simulink model "test_seven_level_flying_cap_leg"  (R2017b)
settings: Solver=ode4  StartTime=0.0  StopTime=0.04  FixedStep=1e-6  MaxStep=1e-4  RelTol=1e-3
libraries: powerlib x10, typhoonHILlib x1
settings Model: Creator=Marcos  LastModifiedBy=Marcos

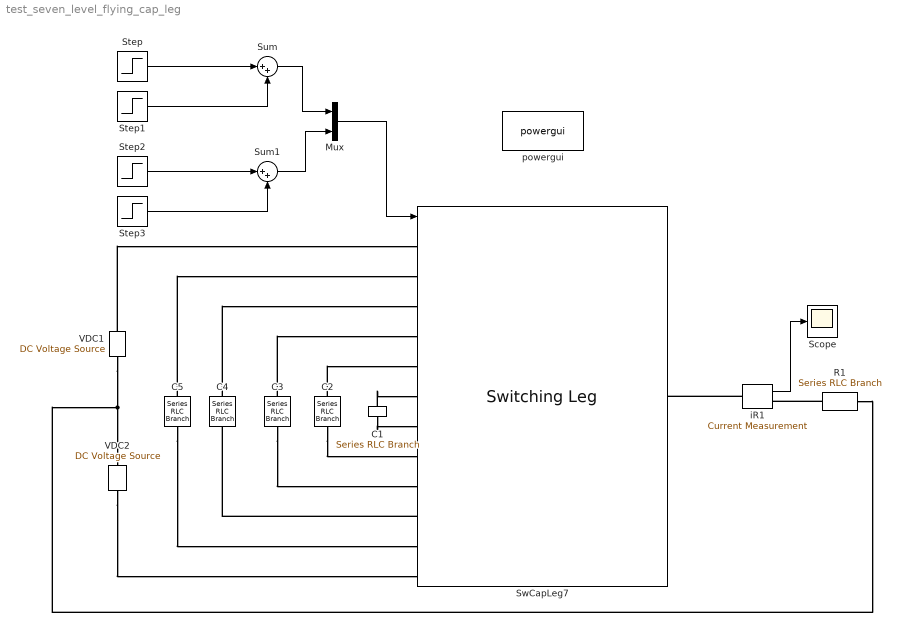
== system test_seven_level_flying_cap_leg ==
  C1 : powerlib/Elements/Series RLC Branch  LConnTagsString=__new0  RConnTagsString=__new0  BranchType=C  Resistance=1  Inductance=1e-3  SetiL0=off  InitialCurrent=0  Capacitance=3e-3  Setx0=on  InitialVoltage=0  Measurements=None
  C{2..5} (4 alike) : powerlib/Elements/Series RLC Branch  LConnTagsString=__new0  RConnTagsString=__new0  BranchType=C  Resistance=1  Inductance=1e-3  SetiL0=off  InitialCurrent=0  Capacitance=1e-3  Setx0=on  InitialVoltage=0  Measurements=None
  Mux : Mux  Inputs=2
  R1 : powerlib/Elements/Series RLC Branch  LConnTagsString=__new0  RConnTagsString=__new0  BranchType=R  Resistance=10  Inductance=1e-3  SetiL0=off  InitialCurrent=0  Capacitance=1e-6  Setx0=off  InitialVoltage=0  Measurements=None
  Scope : Scope
  Step : Step  Time=0  Before=[0 0 0 0 0 0]  After=[0 0 0 0 0 1]  SampleTime=0
  Step1 : Step  Time=0.02  Before=[0 0 0 0 0 0]  After=[1 1 1 1 1 0]  SampleTime=0
  Step2 : Step  Time=0  Before=[0 0 0 0 0 0]  After=[0 1 1 1 1 1]  SampleTime=0
  Step3 : Step  Time=0.02  Before=[0 0 0 0 0 0]  After=[0 -1 -1 -1 -1 -1]  SampleTime=0
  Sum : Sum  Inputs=|++
  Sum1 : Sum  Inputs=|++
  SwCapLeg7 : typhoonHILlib/Switching Leg  LegType=Flying Capacitor  Ttype=on  FCLevels=Seven-level  s1_logic=Active-high  s2_logic=Active-high  s3_logic=Active-high  s4_logic=Active-high  s5_logic=Active-high  s6_logic=Active-high  s7_logic=Active-high  s8_logic=Active-high  s9_logic=Active-high  s10_logic=Active-high  s11_logic=Active-high  s12_logic=Active-high  s13_logic=Active-high  s14_logic=Active-high  s15_logic=Active-high  s16_logic=Active-high  di_s1=1  di_s2=2  di_s3=3  di_s4=4  di_s5=5  di_s6=6  di_s7=7  di_s8=8  di_s9=9  di_s10=10  di_s11=11  di_s12=12  di_s13=13  di_s14=14  di_s15=15  di_s16=16  v_s1=off  v_s2=off  v_s3=off  v_s4=off  v_s5=off  v_s6=off  v_s7=off  v_s8=off  v_s9=off  v_s10=off  v_s11=off  v_s12=off  v_s13=off  v_s14=off  v_s15=off  v_s16=off  i_s1=off  i_s2=off  i_s3=off  i_s4=off  i_s5=off  i_s6=off  i_s7=off  i_s8=off  i_s9=off  i_s10=off  i_s11=off  i_s12=off  i_s13=off  i_s14=off  i_s15=off  i_s16=off  r_on=0.001  v_f=0  r_s=1e4  c_s=inf  toggle_init=on  toggle_draw=on  model_loaded=off  old_pat=typhoonPatterns/FC Leg (7-level)  old_size=250,380
      settings: SourceProductName=Typhoon HIL
  VDC1 : powerlib/Electrical Sources/DC Voltage Source  Amplitude=100  Measurements=None
  VDC2 : powerlib/Electrical Sources/DC Voltage Source  Amplitude=100  Measurements=None
  iR1 : powerlib/Measurements/Current Measurement  PhasorSimulation=off  OutputType=Complex  PSBequivalent=0
  powergui : powerlib/powergui  Priority=1  SimulationMode=Continuous  SampleTime=10e-6  frequency=60  Iterations=50  frequencyindice=0  Pbase=100e6  ErrMax=1e-4  UnitsV=kV  UnitsW=MW  buscounter=0  FunctionMessages=off  echomessages=off  EnableUseOfTLC=off  CurrentSourceSwitches=off  DisableSnubberDevices=off  DisableRonSwitches=off  DisableVfSwitches=off  DisplayEquations=off  SolverType=Tustin/Backward Euler (TBE)  Interpol=off  ExternalGateDelay=off  methode=off  Ts=100  x0status=blocks  SPID=on  SwTol=0  HookPort=off  RestoreLinks=warning  ResistiveCurrentMeasurement=off  Frange=[0:2:500]  Ylog=off  Xlog=on  ShowGrid=off  save=off  variable=ZData  structure=0  ZoomFFT=off  StartTime=0.0  cycles=1  DisplayStyle=1  fundamental=60  FreqAxis=off  MaxFrequency=1000  frequencyindicesteady=1  RmsSteady=1  display=off
  wires:
  iR1/1 -> Scope/1
  Sum/1 -> Mux/1
  Sum1/1 -> Mux/2
  Step/1 -> Sum/1
  Step1/1 -> Sum/2
  Step2/1 -> Sum1/1
  Step3/1 -> Sum1/2
  Mux/1 -> SwCapLeg7/1
  connections:
  R1/LConn1 -- iR1/RConn1
  iR1/LConn1 -- SwCapLeg7/RConn1
  VDC2/LConn1 -- SwCapLeg7/LConn12
  VDC1/RConn1 -- SwCapLeg7/LConn1
  C1/LConn1 -- SwCapLeg7/LConn6
  C1/RConn1 -- SwCapLeg7/LConn7
  C2/LConn1 -- SwCapLeg7/LConn5
  C2/RConn1 -- SwCapLeg7/LConn8
  C3/LConn1 -- SwCapLeg7/LConn4
  C3/RConn1 -- SwCapLeg7/LConn9
  C5/LConn1 -- SwCapLeg7/LConn2
  C5/RConn1 -- SwCapLeg7/LConn11
  SwCapLeg7/LConn10 -- C4/RConn1
  C4/LConn1 -- SwCapLeg7/LConn3
  VDC1/LConn1 -- R1/RConn1 -- VDC2/RConn1
